simulink model "three_axis_gimbal"  (R2017a)
settings: Solver=FixedStepDiscrete  StartTime=0.0  StopTime=10.0  RelTol=1e-3
libraries: simulink x1
settings Model: DataTypeOverride=Off  SimulationMode=external  Creator=mini  LastModifiedBy=mini
settings DataIOCC: SaveOutput=off  SaveTime=off
settings OptimizationCC: BlockReduction=off  ConditionallyExecuteInputs=off  DefaultParameterBehavior=Inlined
settings DebuggingCC: AlgebraicLoopMsg=error  SingleTaskRateTransMsg=error
settings HardwareCC: ProdBitPerPointer=32  ProdBitPerSizeT=32  ProdBitPerPtrDiffT=32  ProdLargestAtomicFloat=None  ProdIntDivRoundTo=Undefined  ProdEndianess=Unspecified  ProdWordSize=32  ProdHWDeviceType=ASIC/FPGA->ASIC/FPGA  ProdEqTarget=off

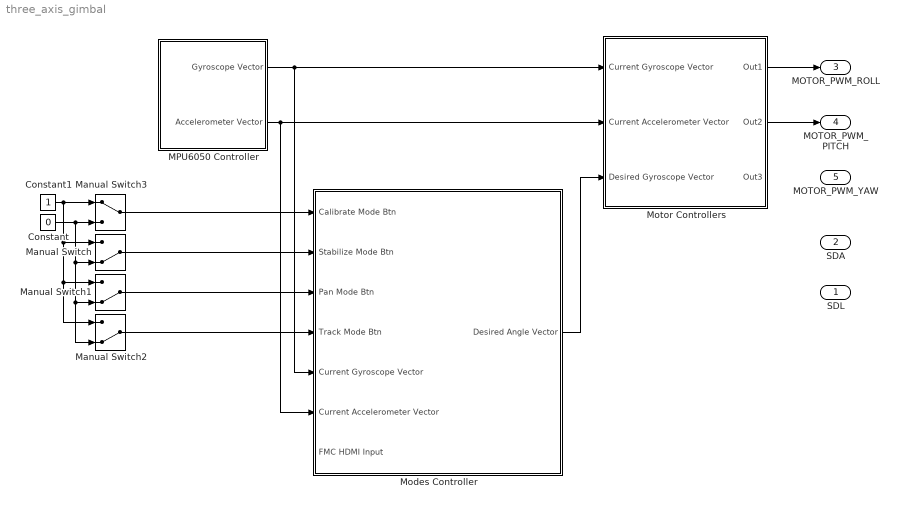
== system three_axis_gimbal ==
  Constant : Constant  Value=0
  Constant1 : Constant
  MPU6050 Controller : Subsystem
  Manual Switch : ManualSwitch  CurrentSetting=0
  Manual Switch1 : ManualSwitch  CurrentSetting=0
  Manual Switch2 : ManualSwitch  CurrentSetting=0
  Manual Switch3 : ManualSwitch
  Modes Controller : Subsystem
  Motor Controllers : Subsystem
  SDL : Outport
  SDA : Outport  Port=2
  MOTOR_PWM_ROLL : Outport  Port=3
  MOTOR_PWM_PITCH : Outport  Port=4
  MOTOR_PWM_YAW : Outport  Port=5
  wires:
  MPU6050 Controller/2(Accelerometer Vector) -> Modes Controller/6(Current Accelerometer Vector), Motor Controllers/2(Current Accelerometer Vector)
  MPU6050 Controller/1(Gyroscope Vector) -> Modes Controller/5(Current Gyroscope Vector), Motor Controllers/1(Current Gyroscope Vector)
  Modes Controller/1(Desired Angle Vector) -> Motor Controllers/3(Desired Gyroscope Vector)
  Manual Switch1/1 -> Modes Controller/3(Pan Mode Btn)
  Manual Switch/1 -> Modes Controller/2(Stabilize Mode Btn)
  Manual Switch2/1 -> Modes Controller/4("Track Mode Btn ")
  Constant1/1 -> Manual Switch3/1, Manual Switch/1, Manual Switch2/1, Manual Switch1/1
  Constant/1 -> Manual Switch3/2, Manual Switch2/2, Manual Switch1/2, Manual Switch/2
  Manual Switch3/1 -> Modes Controller/1(Calibrate Mode Btn)
  Motor Controllers/1(Out1) -> MOTOR_PWM_ROLL/1
  Motor Controllers/2(Out2) -> MOTOR_PWM_PITCH/1

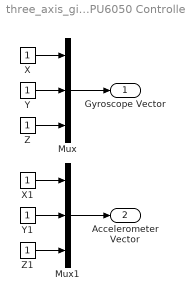
== system three_axis_gimbal/MPU6050 Controller ==
  Mux : Mux  Inputs=3
  Mux1 : Mux  Inputs=3
  X : Constant
  X1 : Constant
  Y : Constant
  Y1 : Constant
  Z : Constant
  Z1 : Constant
  Gyroscope Vector : Outport
  Accelerometer Vector : Outport  Port=2
  wires:
  X/1 -> Mux/1
  Y/1 -> Mux/2
  Z/1 -> Mux/3
  Mux/1 -> Gyroscope Vector/1
  Y1/1 -> Mux1/2
  Z1/1 -> Mux1/3
  X1/1 -> Mux1/1
  Mux1/1 -> Accelerometer Vector/1

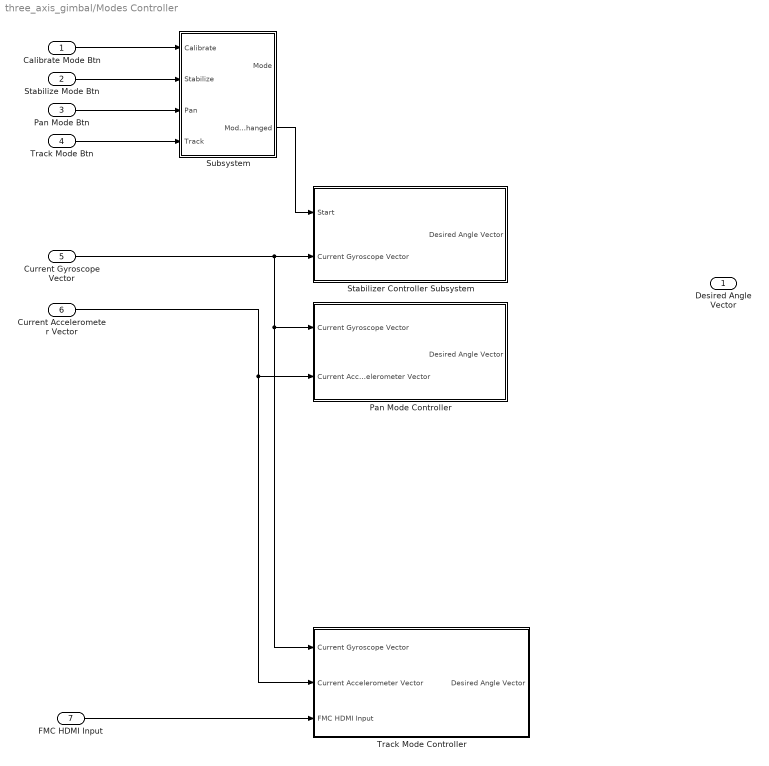
== system three_axis_gimbal/Modes Controller ==
  Calibrate Mode Btn : Inport
  Stabilize Mode Btn : Inport  Port=2
  Pan Mode Btn : Inport  Port=3
  "Track Mode Btn " : Inport  Port=4
  Current Gyroscope Vector : Inport  Port=5
  Current Accelerometer Vector : Inport  Port=6
  FMC HDMI Input : Inport  Port=7
  Pan Mode Controller : Subsystem
  Stabilizer Controller Subsystem : Subsystem
  Subsystem : Subsystem
  Track Mode Controller : Subsystem
  Desired Angle Vector : Outport
  wires:
  Current Gyroscope Vector/1 -> Stabilizer Controller Subsystem/2(Current Gyroscope Vector), Track Mode Controller/1(Current Gyroscope Vector), Pan Mode Controller/1(Current Gyroscope Vector)
  Current Accelerometer Vector/1 -> Track Mode Controller/2(Current Accelerometer Vector), Pan Mode Controller/2(Current Accelerometer Vector)
  FMC HDMI Input/1 -> Track Mode Controller/3(FMC HDMI Input)
  Pan Mode Btn/1 -> Subsystem/3(Pan)
  "Track Mode Btn "/1 -> Subsystem/4(Track)
  Stabilize Mode Btn/1 -> Subsystem/2(Stabilize)
  Calibrate Mode Btn/1 -> Subsystem/1(Calibrate)
  Subsystem/2(Mode Changed) -> Stabilizer Controller Subsystem/1(Start)

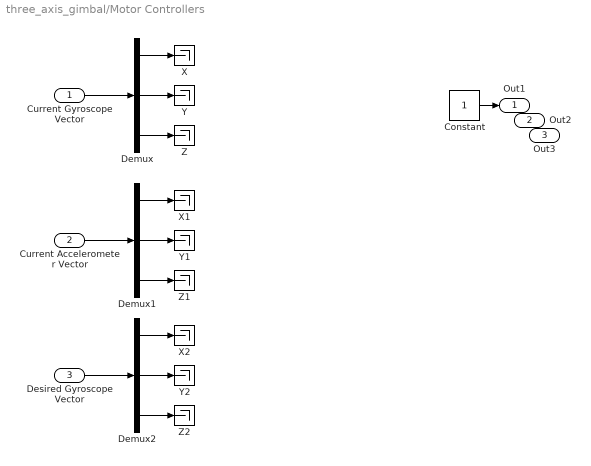
== system three_axis_gimbal/Motor Controllers ==
  Current Gyroscope Vector : Inport
  Current Accelerometer Vector : Inport  Port=2
  Desired Gyroscope Vector : Inport  Port=3
  Constant : Constant
  Demux : Demux  Outputs=3
  Demux1 : Demux  Outputs=3
  Demux2 : Demux  Outputs=3
  X : Terminator
  X1 : Terminator
  X2 : Terminator
  Y : Terminator
  Y1 : Terminator
  Y2 : Terminator
  Z : Terminator
  Z1 : Terminator
  Z2 : Terminator
  Out1 : Outport
  Out2 : Outport  Port=2
  Out3 : Outport  Port=3
  wires:
  Constant/1 -> Out1/1
  Current Gyroscope Vector/1 -> Demux/1
  Demux/1 -> X/1
  Demux/2 -> Y/1
  Demux/3 -> Z/1
  Demux1/2 -> Y1/1
  Current Accelerometer Vector/1 -> Demux1/1
  Demux1/1 -> X1/1
  Demux1/3 -> Z1/1
  Demux2/1 -> X2/1
  Demux2/3 -> Z2/1
  Demux2/2 -> Y2/1
  Desired Gyroscope Vector/1 -> Demux2/1

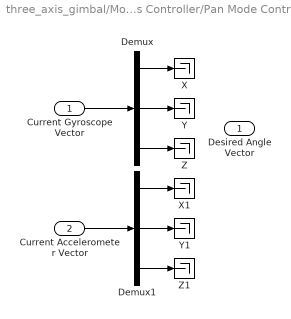
== system three_axis_gimbal/Modes Controller/Pan Mode Controller ==
  Current Gyroscope Vector : Inport
  Current Accelerometer Vector : Inport  Port=2
  Demux : Demux  Outputs=3
  Demux1 : Demux  Outputs=3
  X : Terminator
  X1 : Terminator
  Y : Terminator
  Y1 : Terminator
  Z : Terminator
  Z1 : Terminator
  Desired Angle Vector : Outport
  wires:
  Demux/2 -> Y/1
  Demux/1 -> X/1
  Demux/3 -> Z/1
  Current Gyroscope Vector/1 -> Demux/1
  Demux1/2 -> Y1/1
  Demux1/1 -> X1/1
  Demux1/3 -> Z1/1
  Current Accelerometer Vector/1 -> Demux1/1

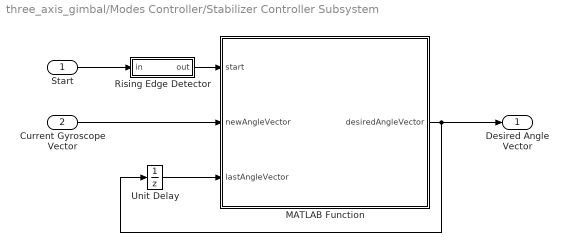
== system three_axis_gimbal/Modes Controller/Stabilizer Controller Subsystem ==
  Start : Inport
  Current Gyroscope Vector : Inport  Port=2
  MATLAB Function : MATLAB Function  TreatAsAtomicUnit=on
  Rising Edge Detector : Subsystem
  Unit Delay : UnitDelay  SampleTime=-1
  Desired Angle Vector : Outport
  wires:
  Unit Delay/1 -> MATLAB Function/3(lastAngleVector)
  MATLAB Function/1(desiredAngleVector) -> Desired Angle Vector/1, Unit Delay/1
  Current Gyroscope Vector/1 -> MATLAB Function/2(newAngleVector)
  Rising Edge Detector/1(out) -> MATLAB Function/1(start)
  Start/1 -> Rising Edge Detector/1(in)

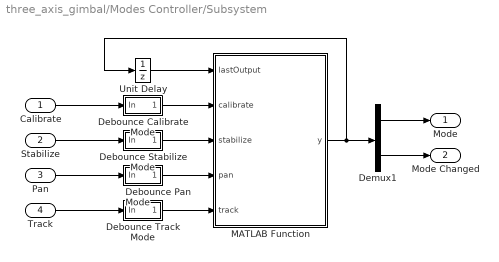
== system three_axis_gimbal/Modes Controller/Subsystem ==
  Calibrate : Inport
  Stabilize : Inport  Port=2
  Pan : Inport  Port=3
  Track : Inport  Port=4
  Debounce Calibrate Mode : Subsystem  TreatAsAtomicUnit=on  mask(Debounce){debounce_count=20}
      mask prompts: debounce_count "Debounce count"
      mask help: Number of consecutive samples before changing states.
  Debounce Pan Mode : Subsystem  TreatAsAtomicUnit=on  mask(Debounce){debounce_count=20}
      mask prompts: debounce_count "Debounce count"
      mask help: Number of consecutive samples before changing states.
  Debounce Stabilize Mode : Subsystem  TreatAsAtomicUnit=on  mask(Debounce){debounce_count=20}
      mask prompts: debounce_count "Debounce count"
      mask help: Number of consecutive samples before changing states.
  Debounce Track Mode : Subsystem  TreatAsAtomicUnit=on  mask(Debounce){debounce_count=20}
      mask prompts: debounce_count "Debounce count"
      mask help: Number of consecutive samples before changing states.
  Demux1 : Demux  Outputs=2
  MATLAB Function : MATLAB Function  TreatAsAtomicUnit=on
  Unit Delay : UnitDelay  SampleTime=-1
  Mode : Outport
  Mode Changed : Outport  Port=2
  wires:
  Pan/1 -> Debounce Pan Mode/1(In)
  Demux1/2 -> Mode Changed/1
  Demux1/1 -> Mode/1
  Calibrate/1 -> Debounce Calibrate Mode/1(In)
  Debounce Pan Mode/1(Out) -> MATLAB Function/4(pan)
  Debounce Track Mode/1(Out) -> MATLAB Function/5(track)
  Unit Delay/1 -> MATLAB Function/1(lastOutput)
  Track/1 -> Debounce Track Mode/1(In)
  Debounce Calibrate Mode/1(Out) -> MATLAB Function/2(calibrate)
  MATLAB Function/1(y) -> Unit Delay/1, Demux1/1
  Debounce Stabilize Mode/1(Out) -> MATLAB Function/3(stabilize)
  Stabilize/1 -> Debounce Stabilize Mode/1(In)

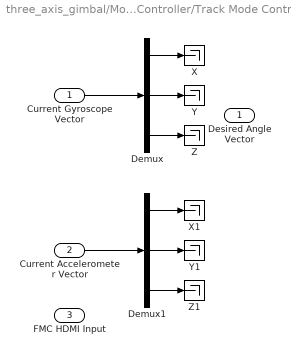
== system three_axis_gimbal/Modes Controller/Track Mode Controller ==
  Current Gyroscope Vector : Inport
  Current Accelerometer Vector : Inport  Port=2
  FMC HDMI Input : Inport  Port=3
  Demux : Demux  Outputs=3
  Demux1 : Demux  Outputs=3
  X : Terminator
  X1 : Terminator
  Y : Terminator
  Y1 : Terminator
  Z : Terminator
  Z1 : Terminator
  Desired Angle Vector : Outport
  wires:
  Demux/2 -> Y/1
  Demux/1 -> X/1
  Demux/3 -> Z/1
  Current Gyroscope Vector/1 -> Demux/1
  Demux1/2 -> Y1/1
  Demux1/1 -> X1/1
  Demux1/3 -> Z1/1
  Current Accelerometer Vector/1 -> Demux1/1

== system three_axis_gimbal/Modes Controller/Stabilizer Controller Subsystem/Rising Edge Detector ==
  in : Inport  OutDataTypeStr=boolean
  Detect Rise Positive : simulink/Logic and Bit Operations/Detect Rise Positive  vinit=0  OutDataTypeStr=boolean
  out : Outport  OutDataTypeStr=boolean
  wires:
  in/1 -> Detect Rise Positive/1
  Detect Rise Positive/1 -> out/1

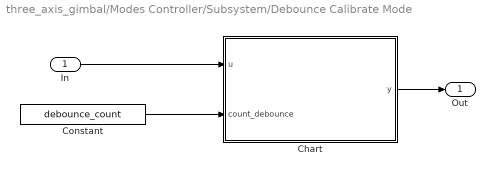
== system three_axis_gimbal/Modes Controller/Subsystem/Debounce Calibrate Mode ==
  In : Inport
  Chart : Stateflow chart  TreatAsAtomicUnit=on
  Constant : Constant  Value=debounce_count  OutDataTypeStr=uint8  SampleTime=-1
  Out : Outport
  wires:
  In/1 -> Chart/1(u)
  Chart/1(y) -> Out/1
  Constant/1 -> Chart/2(count_debounce)

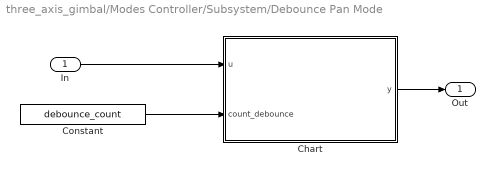
== system three_axis_gimbal/Modes Controller/Subsystem/Debounce Pan Mode ==
  In : Inport
  Chart : Stateflow chart  TreatAsAtomicUnit=on
  Constant : Constant  Value=debounce_count  OutDataTypeStr=uint8  SampleTime=-1
  Out : Outport
  wires:
  In/1 -> Chart/1(u)
  Chart/1(y) -> Out/1
  Constant/1 -> Chart/2(count_debounce)

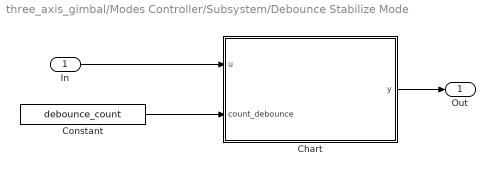
== system three_axis_gimbal/Modes Controller/Subsystem/Debounce Stabilize Mode ==
  In : Inport
  Chart : Stateflow chart  TreatAsAtomicUnit=on
  Constant : Constant  Value=debounce_count  OutDataTypeStr=uint8  SampleTime=-1
  Out : Outport
  wires:
  In/1 -> Chart/1(u)
  Chart/1(y) -> Out/1
  Constant/1 -> Chart/2(count_debounce)

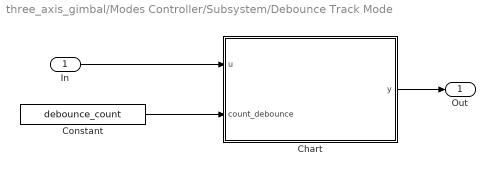
== system three_axis_gimbal/Modes Controller/Subsystem/Debounce Track Mode ==
  In : Inport
  Chart : Stateflow chart  TreatAsAtomicUnit=on
  Constant : Constant  Value=debounce_count  OutDataTypeStr=uint8  SampleTime=-1
  Out : Outport
  wires:
  In/1 -> Chart/1(u)
  Chart/1(y) -> Out/1
  Constant/1 -> Chart/2(count_debounce)

== stateflow chart three_axis_gimbal/Modes Controller/Subsystem/Debounce Calibrate Mode/Chart ==
  settings: executeAtInitialization=1
  (default) -> (junction 2)
  (junction 2) -> (junction 3) [order 1] : [u == u_n1]
  (junction 2) -> (junction 13) [order 2] : {count = 0;}
  (junction 3) -> (junction 5)
  (junction 5) -> (junction 7) [order 1] : [count >= count_debounce]
  (junction 7) -> (junction 9) : {y = u;}
  (junction 5) -> (junction 11) [order 2] : {count = count + 1;}
  (junction 11) -> (junction 13)
  (junction 9) -> (junction 11)
  (junction 13) -> (junction 17) : {u_n1 = u;}
  data: u input; u_n1 local type(u); y output type(u); count local uint8; count_debounce input

== matlab function three_axis_gimbal/Modes Controller/Subsystem/MATLAB Function ==
  data: lastOutput input; y output; calibrate input; stabilize input; pan input; track input
function y = fcn(lastOutput, calibrate, stabilize, pan, track)
    % default action on startup 
    % possible TODO add OFF mode
    
    % won't happen on startup
    if( isvector(lastOutput) && length(lastOutput) == 2 )
        lastMode = lastOutput(1);
        lastUpdated = lastOutput(2);
    else
        % set default mode on startup
        lastMode = 1;
        lastUpdated = 0;
    end
    % change mode based on inputs
    if ( calibrate || lastMode == 0 )
        mode = 1;
    elseif ( stabilize )
        mode = 2;
    elseif ( pan )
        mode = 3;
    elseif ( track )
        mode = 4;
    else
        mode = lastMode;
    end
    % trigger update if mode just changed
    if ( mode ~= lastMode && lastUpdated ~= 1 )
        updated = 1;
    else
        updated = 0;
    end
y = [mode, updated];

== stateflow chart three_axis_gimbal/Modes Controller/Subsystem/Debounce Pan Mode/Chart ==
  settings: executeAtInitialization=1
  (default) -> (junction 2)
  (junction 2) -> (junction 3) [order 1] : [u == u_n1]
  (junction 2) -> (junction 13) [order 2] : {count = 0;}
  (junction 3) -> (junction 5)
  (junction 5) -> (junction 7) [order 1] : [count >= count_debounce]
  (junction 7) -> (junction 9) : {y = u;}
  (junction 5) -> (junction 11) [order 2] : {count = count + 1;}
  (junction 11) -> (junction 13)
  (junction 9) -> (junction 11)
  (junction 13) -> (junction 17) : {u_n1 = u;}
  data: u input; u_n1 local type(u); y output type(u); count local uint8; count_debounce input

== stateflow chart three_axis_gimbal/Modes Controller/Subsystem/Debounce Stabilize Mode/Chart ==
  settings: executeAtInitialization=1
  (default) -> (junction 2)
  (junction 2) -> (junction 3) [order 1] : [u == u_n1]
  (junction 2) -> (junction 13) [order 2] : {count = 0;}
  (junction 3) -> (junction 5)
  (junction 5) -> (junction 7) [order 1] : [count >= count_debounce]
  (junction 7) -> (junction 9) : {y = u;}
  (junction 5) -> (junction 11) [order 2] : {count = count + 1;}
  (junction 11) -> (junction 13)
  (junction 9) -> (junction 11)
  (junction 13) -> (junction 17) : {u_n1 = u;}
  data: u input; u_n1 local type(u); y output type(u); count local uint8; count_debounce input

== stateflow chart three_axis_gimbal/Modes Controller/Subsystem/Debounce Track Mode/Chart ==
  settings: executeAtInitialization=1
  (default) -> (junction 2)
  (junction 2) -> (junction 3) [order 1] : [u == u_n1]
  (junction 2) -> (junction 13) [order 2] : {count = 0;}
  (junction 3) -> (junction 5)
  (junction 5) -> (junction 7) [order 1] : [count >= count_debounce]
  (junction 7) -> (junction 9) : {y = u;}
  (junction 5) -> (junction 11) [order 2] : {count = count + 1;}
  (junction 11) -> (junction 13)
  (junction 9) -> (junction 11)
  (junction 13) -> (junction 17) : {u_n1 = u;}
  data: u input; u_n1 local type(u); y output type(u); count local uint8; count_debounce input

== matlab function three_axis_gimbal/Modes Controller/Stabilizer Controller Subsystem/MATLAB Function ==
  data: start input; newAngleVector input; desiredAngleVector output; lastAngleVector input
function desiredAngleVector = fcn(start, newAngleVector, lastAngleVector)
    % default action on startup 
    if ( start )
        desiredAngleVector = newAngleVector;
    else
        desiredAngleVector = lastAngleVector;
    end
